simulink model "SSM"  (R2022b)
settings: configuration reference "ERT" (kept outside this file)
undefined symbols (not defined in the file): bIsCtl_P, cntPreFailrPerm_C, CodeChkOfsCal_C, DFC, ECM, EiceSilSM, FID, flgIgrDfc_C, nHystFwlAsc_C, nTransFwlAsc_C, Ts_10ms, ubrMax_C, ubrMin_C, uDcLinkPreChrg_C, uThdUmax_C, uThdURng1_C, uThdURng1Hyst_C, uThdURng3Hyst_C
libraries: simulink x8, DSMLib x8
settings Model: Creator=M00039784  LastModifiedBy=M00039784
settings ConfigSetRef: SourceName=ERT  SourceLocation=Base Workspace

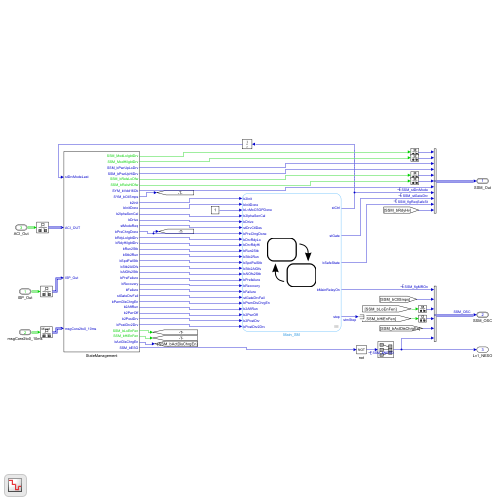
[thumbnail: Simulink's stored preview of the top-level diagram]
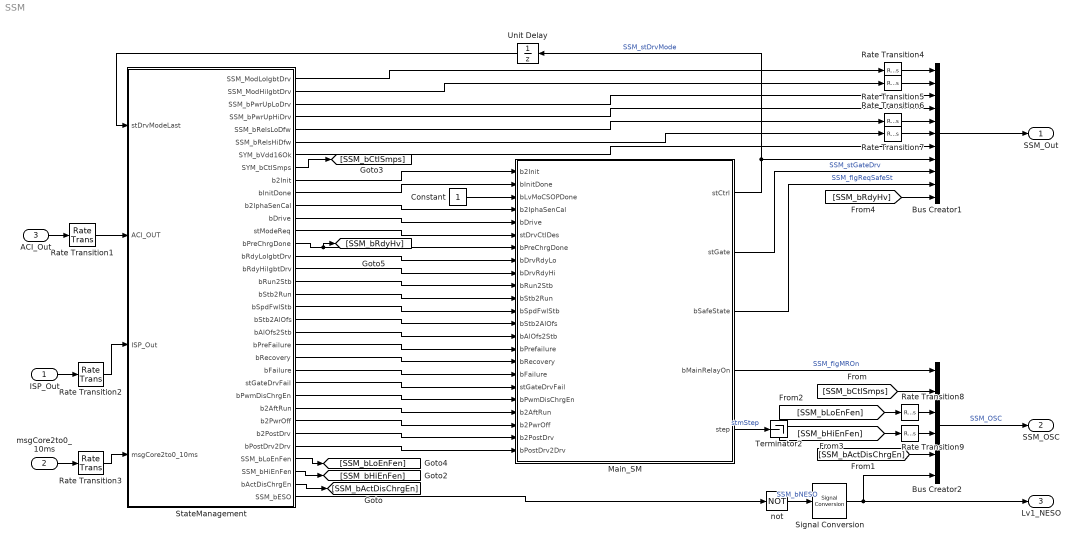
== system SSM ==
  ISP_Out : Inport  OutDataTypeStr=Bus: Core0_ISP_Out
  msgCore2to0_10ms : Inport  Port=2  OutDataTypeStr=Bus: Sig10ms20ST
  ACI_Out : Inport  Port=3  OutDataTypeStr=Bus: IO_In_1ms
  Bus Creator1 : BusCreator  Inputs=11  OutDataTypeStr=Bus: Core0_SSM_Out
  Bus Creator2 : BusCreator  Inputs=6  OutDataTypeStr=Bus: Core0_SSM_OSC
  Constant : Constant  OutDataTypeStr=boolean
  Main_SM : Stateflow chart  Priority=0  TreatAsAtomicUnit=on  SystemSampleTime=Ts_10ms
  Rate Transition{1..9} (9 alike) : RateTransition  OutPortSampleTime=Ts_10ms
  Signal Conversion : SignalConversion  OverrideOpt=off
  StateManagement : Subsystem
  Terminator2 : Terminator
  Unit Delay : UnitDelay  InitialCondition=ECM.Init  SampleTime=-1  HasFrameUpgradeWarning=on
  not : Logic  Operator=NOT  AllPortsSameDT=off  OutDataTypeStr=boolean
  SSM_Out : Outport  OutDataTypeStr=Bus: Core0_SSM_Out  VectorParamsAs1DForOutWhenUnconnected=off
  SSM_OSC : Outport  Port=2  OutDataTypeStr=Bus: Core0_SSM_OSC  VectorParamsAs1DForOutWhenUnconnected=off
  Lv1_NESO : Outport  Port=3  VectorParamsAs1DForOutWhenUnconnected=off
  wires:
  [SSM_bHiEnFen] -> Rate Transition9/1
  Rate Transition6/1 -> Bus Creator1/5
  [SSM_bCtlSmps] -> Bus Creator2/2
  Rate Transition7/1 -> Bus Creator1/6
  StateManagement/33(bActDisChrgEn) -> [SSM_bActDisChrgEn]
  StateManagement/21(bAlOfs2Stb) -> Main_SM/14(bAlOfs2Stb)
  StateManagement/17(bRun2Stb) -> Main_SM/10(bRun2Stb)
  Main_SM/4(bMainRelayOn) -> Bus Creator2/1  "SSM_flgMROn"
  Rate Transition9/1 -> Bus Creator2/4
  Main_SM/5(step) -> Terminator2/1  "stmStep"
  StateManagement/7(SYM_bVdd16Ok) -> Bus Creator1/7
  StateManagement/18(bStb2Run) -> Main_SM/11(bStb2Run)
  StateManagement/25(stGateDrvFail) -> Main_SM/18(stGateDrvFail)
  StateManagement/14(bPreChrgDone) -> [SSM_bRdyHv], Main_SM/7(bPreChrgDone)
  StateManagement/30(bPostDrv2Drv) -> Main_SM/23(bPostDrv2Drv)
  StateManagement/12(bDrive) -> Main_SM/5(bDrive)
  Rate Transition3/1 -> StateManagement/4(msgCore2to0_10ms)
  StateManagement/22(bPreFailure) -> Main_SM/15(bPrefailure)
  Main_SM/3(bSafeState) -> Bus Creator1/10  "SSM_flgReqSafeSt"
  StateManagement/1(SSM_ModLoIgbtDrv) -> Rate Transition4/1
  StateManagement/19(bSpdFwlStb) -> Main_SM/12(bSpdFwlStb)
  Rate Transition1/1 -> StateManagement/2(ACI_OUT)
  StateManagement/31(SSM_bLoEnFen) -> [SSM_bLoEnFen]
  Rate Transition4/1 -> Bus Creator1/1
  StateManagement/9(b2Init) -> Main_SM/1(b2Init)
  StateManagement/24(bFailure) -> Main_SM/17(bFailure)
  StateManagement/28(b2PwrOff) -> Main_SM/21(b2PwrOff)
  ISP_Out/1 -> Rate Transition2/1
  Bus Creator2/1 -> SSM_OSC/1  "SSM_OSC"
  StateManagement/29(b2PostDrv) -> Main_SM/22(b2PostDrv)
  StateManagement/11(b2IphaSenCal) -> Main_SM/4(b2IphaSenCal)
  ACI_Out/1 -> Rate Transition1/1
  Rate Transition5/1 -> Bus Creator1/2
  StateManagement/20(bStb2AlOfs) -> Main_SM/13(bStb2AlOfs)
  StateManagement/16(bRdyHiIgbtDrv) -> Main_SM/9(bDrvRdyHi)
  Bus Creator1/1 -> SSM_Out/1
  Constant/1 -> Main_SM/3(bLvMoCSOPDone)
  StateManagement/5(SSM_bRelsLoDfw) -> Rate Transition6/1
  Rate Transition2/1 -> StateManagement/3(ISP_Out)
  Main_SM/1(stCtrl) -> Unit Delay/1, Bus Creator1/8  "SSM_stDrvMode"
  StateManagement/15(bRdyLoIgbtDrv) -> Main_SM/8(bDrvRdyLo)
  StateManagement/27(b2AftRun) -> Main_SM/20(b2AftRun)
  StateManagement/2(SSM_ModHiIgbtDrv) -> Rate Transition5/1
  [SSM_bLoEnFen] -> Rate Transition8/1
  [SSM_bRdyHv] -> Bus Creator1/11
  StateManagement/8(SYM_bCtlSmps) -> [SSM_bCtlSmps]
  msgCore2to0_10ms/1 -> Rate Transition3/1
  Unit Delay/1 -> StateManagement/1(stDrvModeLast)
  Rate Transition8/1 -> Bus Creator2/3
  StateManagement/23(bRecovery) -> Main_SM/16(bRecovery)
  not/1 -> Signal Conversion/1  "SSM_bNESO"
  StateManagement/32(SSM_bHiEnFen) -> [SSM_bHiEnFen]
  StateManagement/10(bInitDone) -> Main_SM/2(bInitDone)
  [SSM_bActDisChrgEn] -> Bus Creator2/5
  StateManagement/3(SSM_bPwrUpLoDrv) -> Bus Creator1/3
  StateManagement/13(stModeReq) -> Main_SM/6(stDrvCtlDes)
  StateManagement/34(SSM_bESO) -> not/1
  StateManagement/6(SSM_bRelsHiDfw) -> Rate Transition7/1
  StateManagement/4(SSM_bPwrUpHiDrv) -> Bus Creator1/4
  Main_SM/2(stGate) -> Bus Creator1/9  "SSM_stGateDrv"
  StateManagement/26(bPwmDisChrgEn) -> Main_SM/19(bPwmDisChrgEn)
  Signal Conversion/1 -> Lv1_NESO/1, Bus Creator2/6

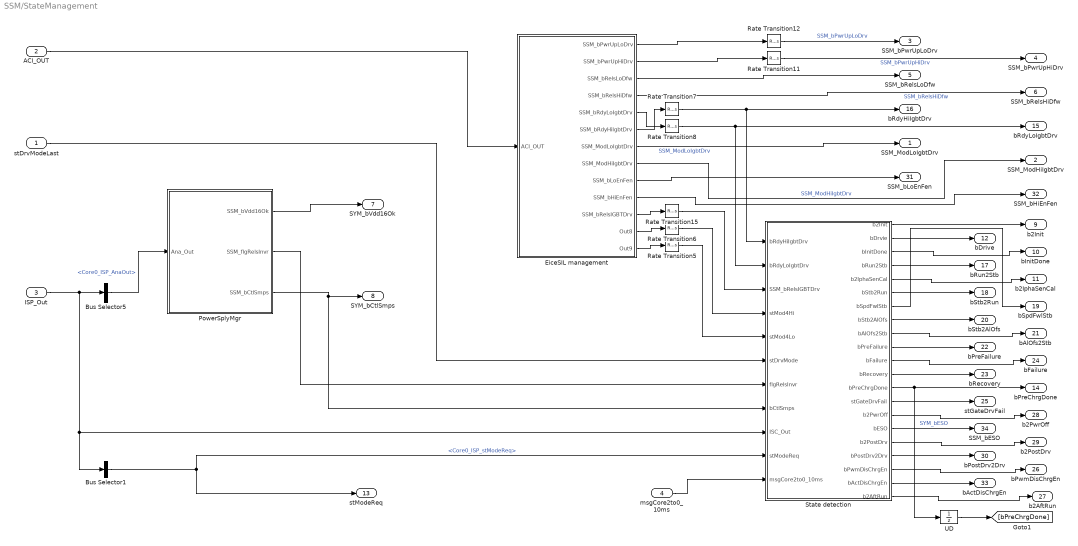
== system SSM/StateManagement ==
  stDrvModeLast : Inport
  ACI_OUT : Inport  Port=2  OutDataTypeStr=Bus: IO_In_1ms
  ISP_Out : Inport  Port=3
  msgCore2to0_10ms : Inport  Port=4
  Bus Selector1 : BusSelector  OutputSignals=Core0_ISP_ComCmd.Core0_ISP_stModeReq
  Bus Selector5 : BusSelector  OutputSignals=Core0_ISP_AnaOut
  EiceSIL management : Subsystem
  PowerSplyMgr : Subsystem
  Rate Transition{5..8,11..12,15} (7 alike) : RateTransition  OutPortSampleTime=Ts_10ms
  State detection : Subsystem
  UD : UnitDelay  SampleTime=-1  HasFrameUpgradeWarning=on
  SSM_ModLoIgbtDrv : Outport  VectorParamsAs1DForOutWhenUnconnected=off
  SSM_ModHiIgbtDrv : Outport  Port=2  VectorParamsAs1DForOutWhenUnconnected=off
  SSM_bPwrUpLoDrv : Outport  Port=3  VectorParamsAs1DForOutWhenUnconnected=off
  SSM_bPwrUpHiDrv : Outport  Port=4  VectorParamsAs1DForOutWhenUnconnected=off
  SSM_bRelsLoDfw : Outport  Port=5  VectorParamsAs1DForOutWhenUnconnected=off
  SSM_bRelsHiDfw : Outport  Port=6  VectorParamsAs1DForOutWhenUnconnected=off
  SYM_bVdd16Ok : Outport  Port=7  VectorParamsAs1DForOutWhenUnconnected=off
  SYM_bCtlSmps : Outport  Port=8  VectorParamsAs1DForOutWhenUnconnected=off
  b2Init : Outport  Port=9  VectorParamsAs1DForOutWhenUnconnected=off
  bInitDone : Outport  Port=10  VectorParamsAs1DForOutWhenUnconnected=off
  b2IphaSenCal : Outport  Port=11  VectorParamsAs1DForOutWhenUnconnected=off
  bDrive : Outport  Port=12  VectorParamsAs1DForOutWhenUnconnected=off
  stModeReq : Outport  Port=13  VectorParamsAs1DForOutWhenUnconnected=off
  bPreChrgDone : Outport  Port=14  VectorParamsAs1DForOutWhenUnconnected=off
  bRdyLoIgbtDrv : Outport  Port=15  VectorParamsAs1DForOutWhenUnconnected=off
  bRdyHiIgbtDrv : Outport  Port=16  VectorParamsAs1DForOutWhenUnconnected=off
  bRun2Stb : Outport  Port=17  VectorParamsAs1DForOutWhenUnconnected=off
  bStb2Run : Outport  Port=18  VectorParamsAs1DForOutWhenUnconnected=off
  bSpdFwlStb : Outport  Port=19  VectorParamsAs1DForOutWhenUnconnected=off
  bStb2AlOfs : Outport  Port=20  VectorParamsAs1DForOutWhenUnconnected=off
  bAlOfs2Stb : Outport  Port=21  VectorParamsAs1DForOutWhenUnconnected=off
  bPreFailure : Outport  Port=22  VectorParamsAs1DForOutWhenUnconnected=off
  bRecovery : Outport  Port=23  VectorParamsAs1DForOutWhenUnconnected=off
  bFailure : Outport  Port=24  VectorParamsAs1DForOutWhenUnconnected=off
  stGateDrvFail : Outport  Port=25  VectorParamsAs1DForOutWhenUnconnected=off
  bPwmDisChrgEn : Outport  Port=26  VectorParamsAs1DForOutWhenUnconnected=off
  b2AftRun : Outport  Port=27  VectorParamsAs1DForOutWhenUnconnected=off
  b2PwrOff : Outport  Port=28  VectorParamsAs1DForOutWhenUnconnected=off
  b2PostDrv : Outport  Port=29  VectorParamsAs1DForOutWhenUnconnected=off
  bPostDrv2Drv : Outport  Port=30  VectorParamsAs1DForOutWhenUnconnected=off
  SSM_bLoEnFen : Outport  Port=31  VectorParamsAs1DForOutWhenUnconnected=off
  SSM_bHiEnFen : Outport  Port=32  VectorParamsAs1DForOutWhenUnconnected=off
  bActDisChrgEn : Outport  Port=33  VectorParamsAs1DForOutWhenUnconnected=off
  SSM_bESO : Outport  Port=34  VectorParamsAs1DForOutWhenUnconnected=off
  wires:
  Bus Selector5/1 -> PowerSplyMgr/1(Ana_Out)  "<Core0_ISP_AnaOut>"
  Bus Selector1/1 -> State detection/10(stModeReq), stModeReq/1  "<Core0_ISP_stModeReq>"
  ISP_Out/1 -> Bus Selector5/1, Bus Selector1/1, State detection/9(ISC_Out)
  PowerSplyMgr/3(SSM_bCtlSmps) -> State detection/8(bCtlSmps), SYM_bCtlSmps/1
  msgCore2to0_10ms/1 -> State detection/11(msgCore2to0_10ms)
  EiceSIL management/1(SSM_bPwrUpLoDrv) -> Rate Transition12/1
  EiceSIL management/2(SSM_bPwrUpHiDrv) -> Rate Transition11/1
  stDrvModeLast/1 -> State detection/6(stDrvMode)
  PowerSplyMgr/1(SSM_bVdd16Ok) -> SYM_bVdd16Ok/1
  EiceSIL management/9(SSM_bLoEnFen) -> SSM_bLoEnFen/1
  EiceSIL management/10(SSM_bHiEnFen) -> SSM_bHiEnFen/1
  State detection/13(bPreChrgDone) -> UD/1, bPreChrgDone/1
  State detection/4(bRun2Stb) -> bRun2Stb/1
  State detection/6(bStb2Run) -> bStb2Run/1
  State detection/7(bSpdFwlStb) -> bSpdFwlStb/1
  State detection/8(bStb2AlOfs) -> bStb2AlOfs/1
  State detection/9(bAlOfs2Stb) -> bAlOfs2Stb/1
  State detection/10(bPreFailure) -> bPreFailure/1
  State detection/12(bRecovery) -> bRecovery/1
  State detection/11(bFailure) -> bFailure/1
  State detection/3(bInitDone) -> bInitDone/1
  State detection/2(bDrvie) -> bDrive/1
  EiceSIL management/12(Out8) -> Rate Transition6/1
  Rate Transition5/1 -> State detection/5(stMod4Lo)
  Rate Transition6/1 -> State detection/4(stMod4Hi)
  EiceSIL management/6(SSM_bRdyHiIgbtDrv) -> Rate Transition7/1
  EiceSIL management/5(SSM_bRdyLoIgbtDrv) -> Rate Transition8/1
  EiceSIL management/4(SSM_bRelsHiDfw) -> SSM_bRelsHiDfw/1  "SSM_bRelsHiDfw"
  Rate Transition11/1 -> SSM_bPwrUpHiDrv/1  "SSM_bPwrUpHiDrv"
  Rate Transition12/1 -> SSM_bPwrUpLoDrv/1  "SSM_bPwrUpLoDrv"
  Rate Transition7/1 -> bRdyHiIgbtDrv/1, State detection/1(bRdyHiIgbtDrv)
  Rate Transition8/1 -> bRdyLoIgbtDrv/1, State detection/2(bRdyLoIgbtDrv)
  EiceSIL management/7(SSM_ModLoIgbtDrv) -> SSM_ModLoIgbtDrv/1  "SSM_ModLoIgbtDrv"
  EiceSIL management/8(SSM_ModHiIgbtDrv) -> SSM_ModHiIgbtDrv/1  "SSM_ModHiIgbtDrv"
  ACI_OUT/1 -> EiceSIL management/1(ACI_OUT)
  EiceSIL management/11(SSM_bRelsIGBTDrv) -> Rate Transition15/1
  Rate Transition15/1 -> State detection/3(SSM_bRelsIGBTDrv)
  UD/1 -> [bPreChrgDone]
  PowerSplyMgr/2(SSM_flgRelsInvr) -> State detection/7(flgRelsInvr)
  State detection/14(stGateDrvFail) -> stGateDrvFail/1
  State detection/16(bESO) -> SSM_bESO/1  "SYM_bESO"
  State detection/5(b2IphaSenCal) -> b2IphaSenCal/1
  State detection/1(b2Init) -> b2Init/1
  State detection/17(b2PostDrv) -> b2PostDrv/1
  State detection/18(bPostDrv2Drv) -> bPostDrv2Drv/1
  State detection/21(b2AftRun) -> b2AftRun/1
  State detection/19(bPwmDisChrgEn) -> bPwmDisChrgEn/1
  State detection/15(b2PwrOff) -> b2PwrOff/1
  State detection/20(bActDisChrgEn) -> bActDisChrgEn/1
  EiceSIL management/13(Out9) -> Rate Transition5/1
  EiceSIL management/3(SSM_bRelsLoDfw) -> SSM_bRelsLoDfw/1

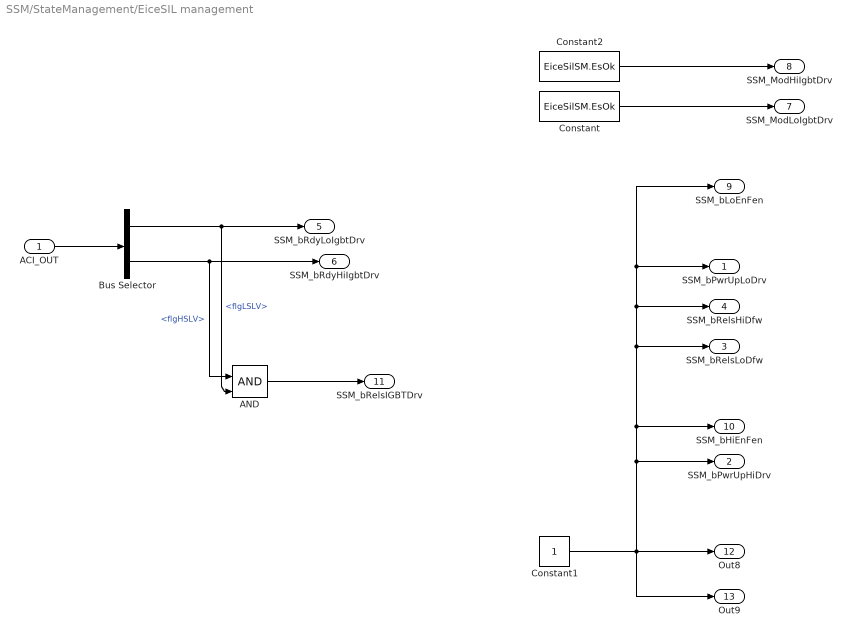
== system SSM/StateManagement/EiceSIL management ==
  ACI_OUT : Inport
  AND : Logic  IconShape=distinctive  AllPortsSameDT=off  OutDataTypeStr=boolean
  Bus Selector : BusSelector  OutputSignals=flgLSLV,flgHSLV
  Constant : Constant  Value=EiceSilSM.EsOk
  Constant1 : Constant  OutDataTypeStr=boolean
  Constant2 : Constant  Value=EiceSilSM.EsOk
  SSM_bPwrUpLoDrv : Outport
  SSM_bPwrUpHiDrv : Outport  Port=2
  SSM_bRelsLoDfw : Outport  Port=3
  SSM_bRelsHiDfw : Outport  Port=4
  SSM_bRdyLoIgbtDrv : Outport  Port=5  VectorParamsAs1DForOutWhenUnconnected=off
  SSM_bRdyHiIgbtDrv : Outport  Port=6  VectorParamsAs1DForOutWhenUnconnected=off
  SSM_ModLoIgbtDrv : Outport  Port=7  VectorParamsAs1DForOutWhenUnconnected=off
  SSM_ModHiIgbtDrv : Outport  Port=8  VectorParamsAs1DForOutWhenUnconnected=off
  SSM_bLoEnFen : Outport  Port=9  VectorParamsAs1DForOutWhenUnconnected=off
  SSM_bHiEnFen : Outport  Port=10  VectorParamsAs1DForOutWhenUnconnected=off
  SSM_bRelsIGBTDrv : Outport  Port=11  VectorParamsAs1DForOutWhenUnconnected=off
  Out8 : Outport  Port=12
  Out9 : Outport  Port=13
  wires:
  Constant/1 -> SSM_ModLoIgbtDrv/1
  Constant1/1 -> SSM_bPwrUpHiDrv/1, SSM_bRelsLoDfw/1, SSM_bRelsHiDfw/1, SSM_bPwrUpLoDrv/1, SSM_bLoEnFen/1, SSM_bHiEnFen/1, Out9/1, Out8/1
  ACI_OUT/1 -> Bus Selector/1
  Bus Selector/1 -> AND/2, SSM_bRdyLoIgbtDrv/1  "<flgLSLV>"
  Bus Selector/2 -> SSM_bRdyHiIgbtDrv/1, AND/1  "<flgHSLV>"
  AND/1 -> SSM_bRelsIGBTDrv/1
  Constant2/1 -> SSM_ModHiIgbtDrv/1

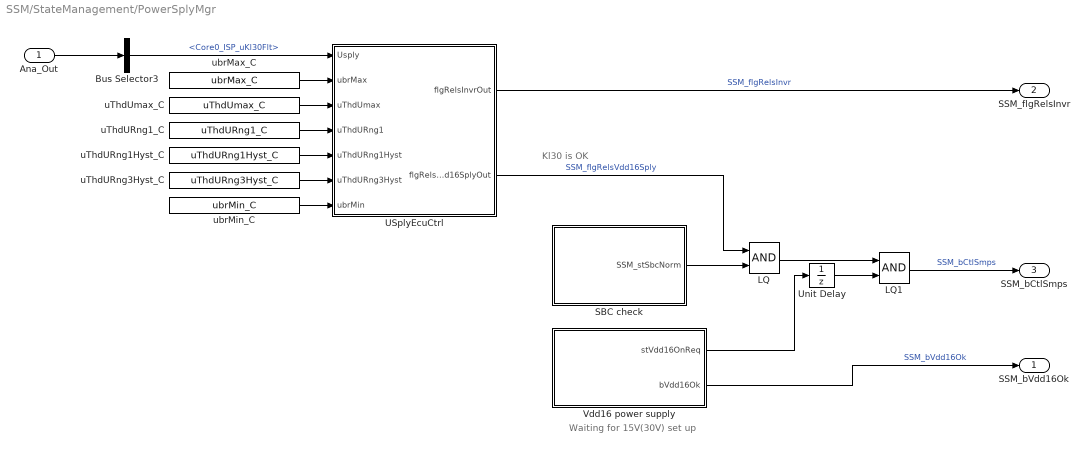
== system SSM/StateManagement/PowerSplyMgr ==
  note: Waiting for 15V(30V) set up
  note: Kl30 is OK
  Ana_Out : Inport
  Bus Selector3 : BusSelector  OutputSignals=Core0_ISP_uKl30Flt
  LQ : Logic  AllPortsSameDT=off  OutDataTypeStr=boolean
  LQ1 : Logic  AllPortsSameDT=off  OutDataTypeStr=boolean
  SBC check : Subsystem
  USplyEcuCtrl : MATLAB Function
  Unit Delay : UnitDelay  InitialCondition=false  SampleTime=-1  HasFrameUpgradeWarning=on
  Vdd16 power supply : Subsystem
  uThdURng1Hyst_C : Constant  Value=uThdURng1Hyst_C
      mask Display:
      | tmpx = get_param(gcbh,'Value');
      | a= evalin('base',[tmpx,'.Value;']);
      | disp([tmpx,': ',num2str(a)]);
  uThdURng1_C : Constant  Value=uThdURng1_C
      mask Display:
      | tmpx = get_param(gcbh,'Value');
      | a= evalin('base',[tmpx,'.Value;']);
      | disp([tmpx,': ',num2str(a)]);
  uThdURng3Hyst_C : Constant  Value=uThdURng3Hyst_C
      mask Display:
      | tmpx = get_param(gcbh,'Value');
      | a= evalin('base',[tmpx,'.Value;']);
      | disp([tmpx,': ',num2str(a)]);
  uThdUmax_C : Constant  Value=uThdUmax_C
      mask Display:
      | tmpx = get_param(gcbh,'Value');
      | a= evalin('base',[tmpx,'.Value;']);
      | disp([tmpx,': ',num2str(a)]);
  ubrMax_C : Constant  Value=ubrMax_C
      mask Display:
      | tmpx = get_param(gcbh,'Value');
      | a= evalin('base',[tmpx,'.Value;']);
      | disp([tmpx,': ',num2str(a)]);
  ubrMin_C : Constant  Value=ubrMin_C
      mask Display:
      | tmpx = get_param(gcbh,'Value');
      | a= evalin('base',[tmpx,'.Value;']);
      | disp([tmpx,': ',num2str(a)]);
  SSM_bVdd16Ok : Outport  VectorParamsAs1DForOutWhenUnconnected=off
  SSM_flgRelsInvr : Outport  Port=2  VectorParamsAs1DForOutWhenUnconnected=off
  SSM_bCtlSmps : Outport  Port=3  VectorParamsAs1DForOutWhenUnconnected=off
  wires:
  Ana_Out/1 -> Bus Selector3/1
  Bus Selector3/1 -> USplyEcuCtrl/1(Usply)  "<Core0_ISP_uKl30Flt>"
  USplyEcuCtrl/1(flgRelsInvrOut) -> SSM_flgRelsInvr/1  "SSM_flgRelsInvr"
  USplyEcuCtrl/2(flgRelsVdd16SplyOut) -> LQ/1  "SSM_flgRelsVdd16Sply"
  SBC check/1(SSM_stSbcNorm) -> LQ/2
  Vdd16 power supply/2(bVdd16Ok) -> SSM_bVdd16Ok/1  "SSM_bVdd16Ok"
  ubrMax_C/1 -> USplyEcuCtrl/2(ubrMax)
  uThdUmax_C/1 -> USplyEcuCtrl/3(uThdUmax)
  uThdURng1_C/1 -> USplyEcuCtrl/4(uThdURng1)
  uThdURng1Hyst_C/1 -> USplyEcuCtrl/5(uThdURng1Hyst)
  uThdURng3Hyst_C/1 -> USplyEcuCtrl/6(uThdURng3Hyst)
  ubrMin_C/1 -> USplyEcuCtrl/7(ubrMin)
  LQ/1 -> LQ1/1
  Vdd16 power supply/1(stVdd16OnReq) -> Unit Delay/1
  Unit Delay/1 -> LQ1/2
  LQ1/1 -> SSM_bCtlSmps/1  "SSM_bCtlSmps"

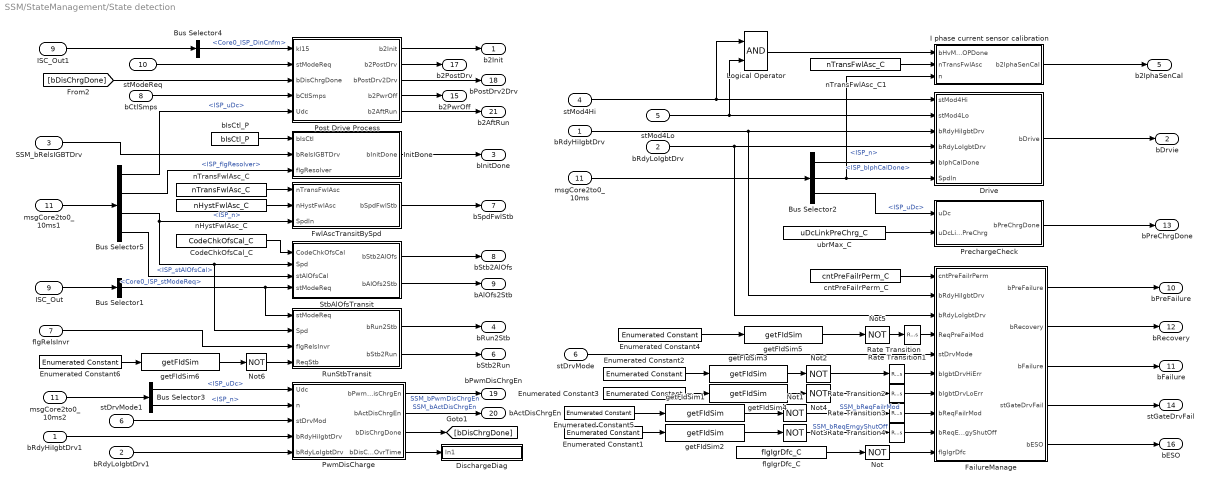
== system SSM/StateManagement/State detection ==
  bRdyHiIgbtDrv : Inport
  bRdyLoIgbtDrv : Inport  Port=2
  SSM_bRelsIGBTDrv : Inport  Port=3
  stMod4Hi : Inport  Port=4
  stMod4Lo : Inport  Port=5
  stDrvMode : Inport  Port=6
  flgRelsInvr : Inport  Port=7
  bCtlSmps : Inport  Port=8
  ISC_Out : Inport  Port=9
  stModeReq : Inport  Port=10
  msgCore2to0_10ms : Inport  Port=11
  Bus Selector1 : BusSelector  OutputSignals=Core0_ISP_ComCmd.Core0_ISP_stModeReq
  Bus Selector2 : BusSelector  OutputSignals=ISP_bIphCalDone,ISP_n,ISP_uDc
  Bus Selector3 : BusSelector  OutputSignals=ISP_uDc,ISP_n
  Bus Selector4 : BusSelector  OutputSignals=Core0_ISP_DinCnfm
  Bus Selector5 : BusSelector  OutputSignals=ISP_uDc,ISP_flgResolver,ISP_n,ISP_stAlOfsCal
  CodeChkOfsCal_C : Constant  Value=CodeChkOfsCal_C
      mask Display:
      | tmpx = get_param(gcbh,'Value');
      | a= evalin('base',[tmpx,'.Value;']);
      | disp([tmpx,': ',num2str(a)]);
  DischargeDiag : Subsystem
  Drive : MATLAB Function
  Enumerated Constant1 : simulink/Sources/Enumerated Constant  OutDataTypeStr=Enum: FID  Value=FID.ReqEmgyShutOff  SampleTime=inf
  Enumerated Constant2 : simulink/Sources/Enumerated Constant  OutDataTypeStr=Enum: FID  Value=FID.ReqIgbtDrvHiInvld  SampleTime=inf
  Enumerated Constant3 : simulink/Sources/Enumerated Constant  OutDataTypeStr=Enum: FID  Value=FID.ReqIgbtDrvLoInvld  SampleTime=inf
  Enumerated Constant4 : simulink/Sources/Enumerated Constant  OutDataTypeStr=Enum: FID  Value=FID.ReqPreFaiMod  SampleTime=inf
  Enumerated Constant5 : simulink/Sources/Enumerated Constant  OutDataTypeStr=Enum: FID  Value=FID.ReqFailrMod  SampleTime=inf
  Enumerated Constant6 : simulink/Sources/Enumerated Constant  OutDataTypeStr=Enum: FID  Value=FID.ReqStandby  SampleTime=inf
  FailureManage : MATLAB Function
  FwlAscTransitBySpd : MATLAB Function
  I phase current sensor calibration : MATLAB Function
  ISC_Out1 : InportShadow  Port=9
  InitDone : MATLAB Function
  Logical Operator : Logic  AllPortsSameDT=off  OutDataTypeStr=boolean
  Not{,1..6} (7 alike) : Logic  Operator=NOT  AllPortsSameDT=off  OutDataTypeStr=boolean
  Post Drive Process : MATLAB Function
  PrechargeCheck : MATLAB Function
  PwmDisCharge : MATLAB Function
  Rate Transition{,1..4} (5 alike) : RateTransition  OutPortSampleTime=Ts_10ms
  RunStbTransit : MATLAB Function
  StbAlOfsTransit : MATLAB Function
  bIsCtl_P : Constant  Value=bIsCtl_P
      mask Display:
      | tmpx = get_param(gcbh,'Value');
      | a= evalin('base',[tmpx,'.Value;']);
      | disp([tmpx,': ',num2str(a)]);
  bRdyHiIgbtDrv1 : InportShadow
  bRdyLoIgbtDrv1 : InportShadow  Port=2
  cntPreFailrPerm_C : Constant  Value=cntPreFailrPerm_C
      mask Display:
      | tmpx = get_param(gcbh,'Value');
      | a= evalin('base',[tmpx,'.Value;']);
      | disp([tmpx,': ',num2str(a)]);
  flgIgrDfc_C : Constant  Value=flgIgrDfc_C
      mask Display:
      | tmpx = get_param(gcbh,'Value');
      | a= evalin('base',[tmpx,'.Value;']);
      | disp([tmpx,': ',num2str(a)]);
  getFIdSim{1..6} (6 alike) : DSMLib/getFIdSim  SystemSampleTime=-1  VariantActivationTime=update diagram  Latency=0  AutoFrameSizeCalculation=off
  msgCore2to0_10ms1 : InportShadow  Port=11
  msgCore2to0_10ms2 : InportShadow  Port=11
  nHystFwlAsc_C : Constant  Value=nHystFwlAsc_C
      mask Display:
      | tmpx = get_param(gcbh,'Value');
      | a= evalin('base',[tmpx,'.Value;']);
      | disp([tmpx,': ',num2str(a)]);
  nTransFwlAsc_C : Constant  Value=nTransFwlAsc_C
      mask Display:
      | tmpx = get_param(gcbh,'Value');
      | a= evalin('base',[tmpx,'.Value;']);
      | disp([tmpx,': ',num2str(a)]);
  nTransFwlAsc_C1 : Constant  Value=nTransFwlAsc_C
      mask Display:
      | tmpx = get_param(gcbh,'Value');
      | a= evalin('base',[tmpx,'.Value;']);
      | disp([tmpx,': ',num2str(a)]);
  stDrvMode1 : InportShadow  Port=6
  ubrMax_C : Constant  Value=uDcLinkPreChrg_C
      mask Display:
      | tmpx = get_param(gcbh,'Value');
      | a= evalin('base',[tmpx,'.Value;']);
      | disp([tmpx,': ',num2str(a)]);
  b2Init : Outport  VectorParamsAs1DForOutWhenUnconnected=off
  bDrvie : Outport  Port=2  VectorParamsAs1DForOutWhenUnconnected=off
  bInitDone : Outport  Port=3  VectorParamsAs1DForOutWhenUnconnected=off
  bRun2Stb : Outport  Port=4  VectorParamsAs1DForOutWhenUnconnected=off
  b2IphaSenCal : Outport  Port=5  VectorParamsAs1DForOutWhenUnconnected=off
  bStb2Run : Outport  Port=6  VectorParamsAs1DForOutWhenUnconnected=off
  bSpdFwlStb : Outport  Port=7  VectorParamsAs1DForOutWhenUnconnected=off
  bStb2AlOfs : Outport  Port=8  VectorParamsAs1DForOutWhenUnconnected=off
  bAlOfs2Stb : Outport  Port=9  VectorParamsAs1DForOutWhenUnconnected=off
  bPreFailure : Outport  Port=10  VectorParamsAs1DForOutWhenUnconnected=off
  bFailure : Outport  Port=11  VectorParamsAs1DForOutWhenUnconnected=off
  bRecovery : Outport  Port=12  VectorParamsAs1DForOutWhenUnconnected=off
  bPreChrgDone : Outport  Port=13  VectorParamsAs1DForOutWhenUnconnected=off
  stGateDrvFail : Outport  Port=14  VectorParamsAs1DForOutWhenUnconnected=off
  b2PwrOff : Outport  Port=15  VectorParamsAs1DForOutWhenUnconnected=off
  bESO : Outport  Port=16  VectorParamsAs1DForOutWhenUnconnected=off
  b2PostDrv : Outport  Port=17  VectorParamsAs1DForOutWhenUnconnected=off
  bPostDrv2Drv : Outport  Port=18  VectorParamsAs1DForOutWhenUnconnected=off
  bPwmDisChrgEn : Outport  Port=19  VectorParamsAs1DForOutWhenUnconnected=off
  bActDisChrgEn : Outport  Port=20  VectorParamsAs1DForOutWhenUnconnected=off
  b2AftRun : Outport  Port=21  VectorParamsAs1DForOutWhenUnconnected=off
  wires:
  Bus Selector5/2 -> InitDone/3(flgResolver)  "<ISP_flgResolver>"
  StbAlOfsTransit/1(bStb2AlOfs) -> bStb2AlOfs/1
  StbAlOfsTransit/2(bAlOfs2Stb) -> bAlOfs2Stb/1
  FailureManage/1(bPreFailure) -> bPreFailure/1
  FailureManage/2(bRecovery) -> bRecovery/1
  FwlAscTransitBySpd/1(bSpdFwlStb) -> bSpdFwlStb/1
  RunStbTransit/2(bStb2Run) -> bStb2Run/1
  RunStbTransit/1(bRun2Stb) -> bRun2Stb/1
  Bus Selector2/3 -> PrechargeCheck/1(uDc)  "<ISP_uDc>"
  Bus Selector2/2 -> I phase current sensor calibration/3(n), Drive/6(SpdIn)  "<ISP_n>"
  bRdyHiIgbtDrv/1 -> FailureManage/2(bRdyHiIgbtDrv), Drive/3(bRdyHiIgbtDrv)
  PrechargeCheck/1(bPreChrgDone) -> bPreChrgDone/1
  Bus Selector2/1 -> Drive/5(bIphCalDone)  "<ISP_bIphCalDone>"
  InitDone/1(bInitDone) -> bInitDone/1
  msgCore2to0_10ms/1 -> Bus Selector2/1
  Bus Selector1/1 -> RunStbTransit/1(stModeReq), StbAlOfsTransit/4(stModeReq)  "<Core0_ISP_stModeReq>"
  stDrvMode/1 -> FailureManage/5(stDrvMode)
  ISC_Out/1 -> Bus Selector1/1
  bRdyLoIgbtDrv/1 -> Drive/4(bRdyLoIgbtDrv), FailureManage/3(bRdyLoIgbtDrv)
  Drive/1(bDrive) -> bDrvie/1
  stMod4Hi/1 -> Logical Operator/1, Drive/1(stMod4Hi)
  stMod4Lo/1 -> Drive/2(stMod4Lo), Logical Operator/2
  SSM_bRelsIGBTDrv/1 -> InitDone/2(bRelsIGBTDrv)
  FailureManage/4(stGateDrvFail) -> stGateDrvFail/1
  FailureManage/5(bESO) -> bESO/1
  Logical Operator/1 -> I phase current sensor calibration/1(bHvMoCSOPDone)
  flgRelsInvr/1 -> RunStbTransit/3(flgRelsInvr)
  msgCore2to0_10ms1/1 -> Bus Selector5/1
  Bus Selector5/3 -> RunStbTransit/2(Spd), StbAlOfsTransit/2(Spd), FwlAscTransitBySpd/3(SpdIn)  "<ISP_n>"
  Bus Selector5/4 -> StbAlOfsTransit/3(stAlOfsCal)  "<ISP_stAlOfsCal>"
  Enumerated Constant5/1 -> getFIdSim1/1
  flgIgrDfc_C/1 -> Not/1
  getFIdSim1/1 -> Not1/1
  Not1/1 -> Rate Transition3/1  "SSM_bReqFailrMod"
  Not/1 -> FailureManage/10(flgIgrDfc)
  FailureManage/3(bFailure) -> bFailure/1
  Enumerated Constant1/1 -> getFIdSim2/1
  getFIdSim2/1 -> Not3/1
  Not3/1 -> Rate Transition4/1  "SSM_bReqEmgyShutOff"
  Enumerated Constant2/1 -> getFIdSim3/1
  Enumerated Constant3/1 -> getFIdSim4/1
  getFIdSim3/1 -> Not2/1
  getFIdSim4/1 -> Not4/1
  Not2/1 -> Rate Transition1/1
  Not4/1 -> Rate Transition2/1
  Not5/1 -> Rate Transition/1
  getFIdSim5/1 -> Not5/1
  Enumerated Constant4/1 -> getFIdSim5/1
  cntPreFailrPerm_C/1 -> FailureManage/1(cntPreFailrPerm)
  getFIdSim6/1 -> Not6/1
  Enumerated Constant6/1 -> getFIdSim6/1
  Not6/1 -> RunStbTransit/4(ReqStb)
  ISC_Out1/1 -> Bus Selector4/1
  Post Drive Process/2(b2PostDrv) -> b2PostDrv/1
  msgCore2to0_10ms2/1 -> Bus Selector3/1
  PwmDisCharge/1(bPwmDisChrgEn) -> bPwmDisChrgEn/1  "SSM_bPwmDisChrgEn"
  Bus Selector3/1 -> PwmDisCharge/1(Udc)  "<ISP_uDc>"
  stDrvMode1/1 -> PwmDisCharge/3(stDrvMod)
  bRdyHiIgbtDrv1/1 -> PwmDisCharge/4(bRdyHiIgbtDrv)
  bRdyLoIgbtDrv1/1 -> PwmDisCharge/5(bRdyLoIgbtDrv)
  Bus Selector3/2 -> PwmDisCharge/2(n)  "<ISP_n>"
  PwmDisCharge/4(bDisChrgOvrTime) -> DischargeDiag/1(In1)
  Post Drive Process/1(b2Init) -> b2Init/1
  Post Drive Process/3(bPostDrv2Drv) -> bPostDrv2Drv/1
  Bus Selector4/1 -> Post Drive Process/1(kl15)  "<Core0_ISP_DinCnfm>"
  stModeReq/1 -> Post Drive Process/2(stModeReq)
  PwmDisCharge/3(bDisChrgDone) -> [bDisChrgDone]
  [bDisChrgDone] -> Post Drive Process/3(bDisChrgDone)
  I phase current sensor calibration/1(b2IphaSenCal) -> b2IphaSenCal/1
  nTransFwlAsc_C/1 -> FwlAscTransitBySpd/1(nTransFwlAsc)
  nHystFwlAsc_C/1 -> FwlAscTransitBySpd/2(nHystFwlAsc)
  nTransFwlAsc_C1/1 -> I phase current sensor calibration/2(nTransFwlAsc)
  Post Drive Process/4(b2PwrOff) -> b2PwrOff/1
  Post Drive Process/5(b2AftRun) -> b2AftRun/1
  bCtlSmps/1 -> Post Drive Process/4(bCtlSmps)
  ubrMax_C/1 -> PrechargeCheck/2(uDcLinkPreChrg)
  CodeChkOfsCal_C/1 -> StbAlOfsTransit/1(CodeChkOfsCal)
  PwmDisCharge/2(bActDisChrgEn) -> bActDisChrgEn/1  "SSM_bActDisChrgEn"
  Bus Selector5/1 -> Post Drive Process/5(Udc)  "<ISP_uDc>"
  bIsCtl_P/1 -> InitDone/1(bIsCtl)
  Rate Transition/1 -> FailureManage/4(ReqPreFaiMod)
  Rate Transition1/1 -> FailureManage/6(bIgbtDrvHiErr)
  Rate Transition2/1 -> FailureManage/7(bIgbtDrvLoErr)
  Rate Transition3/1 -> FailureManage/8(bReqFailrMod)
  Rate Transition4/1 -> FailureManage/9(bReqEmgyShutOff)

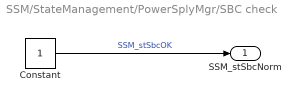
== system SSM/StateManagement/PowerSplyMgr/SBC check ==
  Constant : Constant  OutDataTypeStr=boolean
  SSM_stSbcNorm : Outport  VectorParamsAs1DForOutWhenUnconnected=off
  wires:
  Constant/1 -> SSM_stSbcNorm/1  "SSM_stSbcOK"

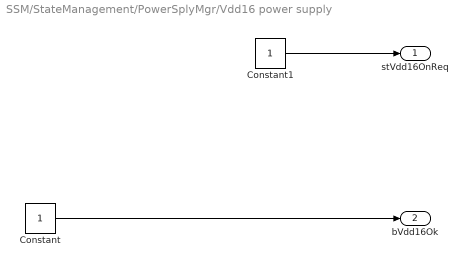
== system SSM/StateManagement/PowerSplyMgr/Vdd16 power supply ==
  Constant : Constant  OutDataTypeStr=boolean
  Constant1 : Constant  OutDataTypeStr=boolean
  stVdd16OnReq : Outport  VectorParamsAs1DForOutWhenUnconnected=off
  bVdd16Ok : Outport  Port=2  VectorParamsAs1DForOutWhenUnconnected=off
  wires:
  Constant/1 -> bVdd16Ok/1
  Constant1/1 -> stVdd16OnReq/1

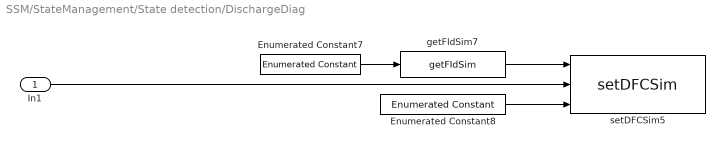
== system SSM/StateManagement/State detection/DischargeDiag ==
  In1 : Inport
  Enumerated Constant7 : simulink/Sources/Enumerated Constant  OutDataTypeStr=Enum: FID  Value=FID.DiagUdcDisChrg  SampleTime=inf
  Enumerated Constant8 : simulink/Sources/Enumerated Constant  OutDataTypeStr=Enum: DFC  Value=DFC.UdcDisChrgOvrTime  SampleTime=inf
  getFIdSim7 : DSMLib/getFIdSim  SystemSampleTime=-1  VariantActivationTime=update diagram  Latency=0  AutoFrameSizeCalculation=off
  setDFCSim5 : DSMLib/setDFCSim  SystemSampleTime=-1  VariantActivationTime=update diagram  Latency=0  AutoFrameSizeCalculation=off
  wires:
  In1/1 -> setDFCSim5/2
  Enumerated Constant7/1 -> getFIdSim7/1
  getFIdSim7/1 -> setDFCSim5/1
  Enumerated Constant8/1 -> setDFCSim5/3

== stateflow chart SSM/Main_SM ==
  state PreDrive
    en: %predrive init
    state State_PreInit
      en:step = 0;
      stCtrl = ECM.PreInit;
      bSafeState = true;
      stGate = EGM.Freewheel;
      bPreDrvDone = false;
    state State_Init
      en:step = 1;
      bSafeState = true;
      stCtrl = ECM.Init;
      stGate = EGM.Freewheel;
      bMainRelayOn = true; %MR on
    state State_LVMOCSOP
      en:step = 2;
      bSafeState = true;
      stCtrl =ECM.LvMoCSOP;
      %stGate defined in CddHwMgr
    state State_PREDRVDone
      en:step = 3;
      bSafeState = true;
      stCtrl =ECM.PreDrvDone;
      stGate = EGM.Freewheel;
      bPreDrvDone = true;
    (default) -> State_PreInit
    State_PreInit -> State_Init : [b2Init]
    State_Init -> State_LVMOCSOP : [bInitDone]
    State_LVMOCSOP -> State_PREDRVDone : [bLvMoCSOPDone]
  state PostDrive
    en: % postdrive init
    state State_Discharge
      en:step=11;
      stCtrl = ECM.Discharge;
      stGate = StASC(bDrvRdyLo,bDrvRdyHi);
      du:
      if bPwmDisChrgEn
      stGate = EGM.PWMDischarge;
      else
      stGate = StASC(bDrvRdyLo,bDrvRdyHi);
      end
    state State_PowerOff
      en:step=12;
      stCtrl = ECM.PowerOff;
      stGate = EGM.Freewheel;
    state State_Afterrun
      en:step=12;
      stCtrl = ECM.Afterrun;
      stGate = EGM.Freewheel;
      bMainRelayOn = false;
    (default) -> State_Discharge
    State_Discharge -> State_PowerOff : [b2PwrOff]
    State_PowerOff -> State_Afterrun : [b2AftRun]
  state Drive
    en:% drive init
    state State_Ready
      state State_Run
        en:step=9;
        [stCtrl,stGate] = StRun(stDrvCtlDes);
        du: [stCtrl,stGate] = StRun(stDrvCtlDes);
        ex: stGate = EGM.Freewheel
      state State_Standby
        en:
        step=7;
        bSafeState = false;
        stCtrl = ECM.Standby;
        if bSpdFwlStb
        stGate = EGM.Freewheel;
        else
        stGate = EGM.Freewheel;
        end
        du:
        if bSpdFwlStb
        stGate = EGM.Freewheel;
        else
        stGate = EGM.Freewheel;
        end
      state State_PreFailure
        en:step =10;
        stCtrl = ECM.PreFailure;
        stGate = EGM.Freewheel;
      state State_AlOfsDone
        en:step=8;
        stCtrl = ECM.alOfsCal;
        stGate = EGM.PWMRun;
      State_Run -> State_Standby [order 1] : [bRun2Stb]
      State_Standby -> State_Run [order 1] : [bStb2Run]
      State_Run -> State_PreFailure [order 2] : [bPrefailure]
      (default) -> State_Standby
      State_PreFailure -> State_Standby : [bRecovery]
      State_Standby -> State_AlOfsDone [order 2] : [bStb2AlOfs]
      State_AlOfsDone -> State_Standby : [bAlOfs2Stb]
    state State_PreCharge
      en:step =4;
      bSafeState = true;
      stCtrl = ECM.PreCharge;
      stGate = EGM.Freewheel;
    state State_HVMOCSOP
      en:step =5;
      stCtrl = ECM.HvMoCSOP;
      %stGate defined in CddHwMgr
    state State_SenCal
      en:step =6;
      bSafeState = false;
      stCtrl = ECM.SensCal;
      stGate = EGM.Freewheel;
    (default) -> State_PreCharge
    State_PreCharge -> State_HVMOCSOP : [bPreChrgDone]
    State_HVMOCSOP -> State_SenCal : [b2IphaSenCal]
    State_SenCal -> State_Ready : [bDrive]
  note: Discharge: High voltage (Vdc Link) discharge
      |
      | PwrOff: Low voltage side and IGBT driver power off.
  state State_Failure
    entry:step=12;
    bSafeState = true;
    stCtrl = ECM.Failure;
    stGate =stGateDrvFail;
  (default) -> PreDrive
  PreDrive -> PostDrive [order 1] : [b2PostDrv]
  PostDrive -> Drive : [bPostDrv2Drv]
  PreDrive -> Drive [order 2] : [bPreDrvDone]
  Drive -> PostDrive [order 1] : [b2PostDrv]
  State_Failure -> PostDrive : [b2PostDrv]
  Drive -> State_Failure [order 2] : [bFailure]
  data: des function_input; drv function_output; gate function_output; stIgbtDrvLo function_input; gate function_output; stIgbtDrvHi function_input; stCtrl output; stGate output; b2Init input; bInitDone input boolean; bLvMoCSOPDone input boolean; b2IphaSenCal input boolean; bDrive input boolean; stDrvCtlDes input Enum: ECM; bPreChrgDone input boolean; bDrvRdyLo input boolean; bDrvRdyHi input boolean; bRun2Stb input boolean; bStb2Run input; bSpdFwlStb input boolean; bSkipInit constant boolean =1; bSafeState output boolean; bMainRelayOn output boolean; step output; bStb2AlOfs input; bAlOfs2Stb input; bPrefailure input boolean; bRecovery input boolean; bFailure input boolean; stGateDrvFail input; bPwmDisChrgEn input; b2AftRun input boolean; b2PwrOff input; bPreDrvDone local boolean =false; b2PostDrv input; bPostDrv2Drv input
  function [drv,gate] = StRun(des):
    | function [drv,gate] = StRun(des)
    |     if (des == ECM.TrqCtrl) 
    |         drv = ECM.TrqCtrl;
    |         gate = EGM.PWMRun;
    |     elseif (des == ECM.nCtrl) 
    |         drv = ECM.nCtrl;
    |         gate = EGM.PWMRun;
    |     elseif (des == ECM.UdcCtrl) 
    |         drv = ECM.UdcCtrl;
    |         gate = EGM.PWMRun;
    |     elseif (des == ECM.IFCtrl) 
    |         drv = ECM.IFCtrl;
    |         gate = EGM.PWMRun;
    |     elseif (des == ECM.IsCtrl) 
    |     drv = ECM.IsCtrl;
    |     gate = EGM.PWMRun;
    |     else 
    |         drv = ECM.Standby;
    |         gate = EGM.Freewheel;
    |     end
  function gate  = StASC(stIgbtDrvLo,stIgbtDrvHi):
    | function gate  = StASC(stIgbtDrvLo,stIgbtDrvHi)
    | if (stIgbtDrvLo) 
    |     gate = EGM.Shortcircuit;
    | elseif (stIgbtDrvHi)
    |     gate = EGM.ShortcircuitTop;
    | else
    |     gate = EGM.Freewheel;
    | end

== matlab function SSM/StateManagement/State detection/InitDone ==
  data: bIsCtl input; bRelsIGBTDrv input; bInitDone output; flgResolver input
function bInitDone  = fcn(bIsCtl,bRelsIGBTDrv,flgResolver)
%
bInitDone = bRelsIGBTDrv&&(flgResolver==uint8(2)||bIsCtl);

== matlab function SSM/StateManagement/State detection/Drive ==
  data: stMod4Hi input; stMod4Lo input; bRdyHiIgbtDrv input; bDrive output; bRdyLoIgbtDrv input; bIphCalDone input; SpdIn input
function bDrive  = fcn(stMod4Hi,stMod4Lo,bRdyHiIgbtDrv,bRdyLoIgbtDrv,bIphCalDone,SpdIn)
%

if SpdIn<single(4000)
    if bIphCalDone==true
        bSenCalStb = true;
    else
        bSenCalStb = false;
    end
else
    bSenCalStb= true;
end

bDrive = bRdyHiIgbtDrv&&bRdyLoIgbtDrv&&stMod4Hi&&stMod4Lo&&bSenCalStb;

== matlab function SSM/StateManagement/State detection/PwmDisCharge ==
  data: Udc input; n input; bPwmDisChrgEn output; bActDisChrgEn output; stDrvMod input; bDisChrgDone output; bRdyHiIgbtDrv input; bRdyLoIgbtDrv input; bDisChrgOvrTime output
function [bPwmDisChrgEn,bActDisChrgEn,bDisChrgDone,bDisChrgOvrTime]  = fcn(Udc,n,stDrvMod,bRdyHiIgbtDrv,bRdyLoIgbtDrv)
%
persistent cntDisCharg;
persistent bDisChrgDoneTmp;
persistent bActDisChrgEnTmp;
persistent bDisChrgOvrTimeTmp;

if isempty(cntDisCharg)
    cntDisCharg = uint16(0);
    bDisChrgDoneTmp = false;
    bDisChrgOvrTimeTmp = false;
    bActDisChrgEnTmp = false;
end

if stDrvMod==ECM.Discharge
    cntDisCharg = cntDisCharg + uint16(1);
    
    if Udc<single(55) %<55V
        bDisChrgDoneTmp = true;
    else
        if bRdyHiIgbtDrv&&bRdyLoIgbtDrv&&(abs(n)<single(500))
            bActDisChrgEnTmp = true;
        else
            bActDisChrgEnTmp = false;
        end 
    end
    
    if cntDisCharg>uint16(200) %2s
        cntDisCharg = uint16(201);
        bActDisChrgEnTmp = false;
        bDisChrgOvrTimeTmp = true;
    end
else
    bActDisChrgEnTmp = false;
    bDisChrgDoneTmp = false;
    cntDisCharg = uint16(0);
end

bDisChrgDone = bDisChrgDoneTmp;
bActDisChrgEn = bActDisChrgEnTmp;
bPwmDisChrgEn = false;
bDisChrgOvrTime = bDisChrgOvrTimeTmp;

== matlab function SSM/StateManagement/PowerSplyMgr/USplyEcuCtrl ==
  data: Usply input; ubrMax input; uThdUmax input; flgRelsInvrOut output; uThdURng1 input; uThdURng1Hyst input; uThdURng3Hyst input; ubrMin input; flgRelsVdd16SplyOut output
function [flgRelsInvrOut,flgRelsVdd16SplyOut]  = fcn(Usply,ubrMax,uThdUmax,uThdURng1,uThdURng1Hyst,uThdURng3Hyst,ubrMin)
%
persistent tiDelta;
persistent tiURng1Actv;
persistent tiURng2Actv;
persistent tiURng3Actv;
persistent tiURng4Actv;
persistent flgURng1Actv;
persistent flgURng2Actv;
persistent flgURng3Actv;
persistent tiURng1Rcv_C;
persistent tiURng2Rcv_C;
persistent tiURng3Rcv_C;
persistent tiURng4Rcv_C;
persistent tiMaxRngC_C;
persistent flgRelsInvr;
persistent flgRelsVdd16Sply;

if isempty(tiDelta)
    tiDelta = single(0.01);
    tiURng1Actv = single(0);
    tiURng2Actv = single(0);
    tiURng3Actv = single(0);
    tiURng4Actv = single(0);
    flgURng1Actv = false;
    flgURng2Actv = false;
    flgURng3Actv = false;
    tiURng1Rcv_C = single(0.03);
    tiURng2Rcv_C = single(0.03);
    tiURng3Rcv_C = single(0.03);
    tiURng4Rcv_C = single(0.03);
    tiMaxRngC_C = single(3);
    flgRelsInvr = false;
    flgRelsVdd16Sply = false;
end

%URng1:9V~17V
if Usply>uThdUmax %17V, uThdUmax is about 17V, inverter will work in normal mode
    tiURng4Actv = tiURng4Actv + tiDelta;
    tiURng1Actv = tiURng1Actv - tiDelta;
    
    if tiURng4Actv>tiMaxRngC_C
            tiURng4Actv = tiMaxRngC_C;
    end
    
    if tiURng1Actv<single(0)
        tiURng1Actv = single(0);
    end
    
    flgURng1Actv = false;
else
    if Usply<(uThdUmax-uThdURng1Hyst)% about16.8V  inverter will work in normal mode
        tiURng4Actv = single(0);
        tiURng1Actv = tiURng1Actv + tiDelta;
        
        if tiURng1Actv>tiMaxRngC_C
            tiURng1Actv = tiMaxRngC_C;
        end
        
        flgURng1Actv = true;  %range 9V~17V is true
    end
end

%URng2:6V~9V
if Usply>uThdURng1 % >9V
    tiURng2Actv = tiURng2Actv - tiDelta;
    
    if tiURng2Actv<single(0)
        tiURng2Actv = single(0);
    end
    
    flgURng2Actv = false;
else
    if Usply<(uThdURng1-uThdURng1Hyst) % <8.8V
        tiURng1Actv = single(0);
        tiURng2Actv = tiURng2Actv + tiDelta;
        
        if tiURng2Actv>tiMaxRngC_C
            tiURng2Actv = tiMaxRngC_C;
        end
        
        flgURng2Actv = true;  %range 6V~8V is true
    end
end
    
%URng3:<5.8V
if Usply>(ubrMin+uThdURng3Hyst) % >6V
    tiURng3Actv = tiURng3Actv - tiDelta;
    
    if tiURng3Actv<single(0)
        tiURng3Actv = single(0);
    end
    
    flgURng3Actv = false;
else
    if Usply<ubrMin %5.8V
        tiURng2Actv = single(0);
        tiURng3Actv = tiURng3Actv + tiDelta;
        
        if tiURng3Actv>tiMaxRngC_C
            tiURng3Actv = tiMaxRngC_C;
        end
        
        flgURng3Actv = true;  %range <5.8 is true
    end
end
    
if (tiURng1Actv>tiURng1Rcv_C)&&flgURng1Actv&&(~flgURng2Actv)&&(~flgURng3Actv)
    flgRelsInvr = true;
    flgRelsVdd16Sply = true;
end

%>17V or 6~9V
if ((tiURng2Actv>tiURng2Rcv_C)&&flgURng2Actv&&(~flgURng3Actv))||((tiURng4Actv>tiURng4Rcv_C)&&(~flgURng1Actv))
    flgRelsInvr = false;
    flgRelsVdd16Sply = true;
end

if (Usply>ubrMax)||((tiURng3Actv>tiURng3Rcv_C)&&flgURng3Actv)  %Current maximum is about 22V
    flgRelsInvr = false;
    flgRelsVdd16Sply = false;
end

flgRelsInvrOut = flgRelsInvr;
flgRelsVdd16SplyOut = flgRelsVdd16Sply;

== matlab function SSM/StateManagement/State detection/Post Drive Process ==
  data: kl15 input; b2Init output; b2PostDrv output; bPostDrv2Drv output; stModeReq input; bDisChrgDone input; bCtlSmps input; Udc input; b2PwrOff output; b2AftRun output
function [b2Init,b2PostDrv,bPostDrv2Drv,b2PwrOff,b2AftRun]  = fcn(kl15,stModeReq,bDisChrgDone,bCtlSmps,Udc)
%
b2Init = kl15;
b2PostDrv = (~kl15)||(stModeReq==ECM.Discharge);
bPostDrv2Drv = false;
b2PwrOff = (~kl15)&&(bDisChrgDone||(Udc<single(55)));
b2AftRun = ~bCtlSmps;

== matlab function SSM/StateManagement/State detection/I phase current sensor calibration ==
  data: bHvMoCSOPDone input; nTransFwlAsc input; b2IphaSenCal output; n input
function b2IphaSenCal  = fcn(bHvMoCSOPDone,nTransFwlAsc,n)
%
b2IphaSenCal = bHvMoCSOPDone&&(abs(n)<nTransFwlAsc);

== matlab function SSM/StateManagement/State detection/FwlAscTransitBySpd ==
  data: nTransFwlAsc input; nHystFwlAsc input; SpdIn input; bSpdFwlStb output
function bSpdFwlStb  = fcn(nTransFwlAsc,nHystFwlAsc,SpdIn)
%
persistent flgSpdFwl;

if isempty(flgSpdFwl)
    flgSpdFwl = false;
end

if SpdIn<single(nTransFwlAsc)
    flgSpdFwl = false;
elseif SpdIn>single(nTransFwlAsc+nHystFwlAsc)
    flgSpdFwl = true;   
end

bSpdFwlStb = flgSpdFwl;

== matlab function SSM/StateManagement/State detection/RunStbTransit ==
  data: stModeReq input; Spd input; flgRelsInvr input; ReqStb input; bRun2Stb output; bStb2Run output
function [bRun2Stb,bStb2Run]  = fcn(stModeReq,Spd,flgRelsInvr,ReqStb)
%
nAbs = abs(Spd);
if ReqStb||nAbs>single(19000) %375
    bStb2Run = false;
    bRun2Stb = true;
else
    if ((stModeReq==ECM.TrqCtrl)||(stModeReq==ECM.nCtrl)||(stModeReq==ECM.IFCtrl)||(stModeReq==ECM.UdcCtrl)||(stModeReq==ECM.IsCtrl))...
       &&flgRelsInvr
        bStb2Run = true;
        bRun2Stb = false;
    else
        bStb2Run = false;
        bRun2Stb = true;
    end
end

== matlab function SSM/StateManagement/State detection/StbAlOfsTransit ==
  data: CodeChkOfsCal input; Spd input; stAlOfsCal input; stModeReq input; bStb2AlOfs output; bAlOfs2Stb output
function [bStb2AlOfs,bAlOfs2Stb]  = fcn(CodeChkOfsCal,Spd,stAlOfsCal,stModeReq)
%
%stAlOfsCal:
%0: Init or rotor position offset calibration processing
%1: Rotor position offset calibration successed
%2: Rotor position offset calibration failed
bStb2AlOfs = (stModeReq==ECM.alOfsCal)&&(stAlOfsCal==uint8(0))&&(Spd<single(100))&&(CodeChkOfsCal==uint32(12345678));

bAlOfs2Stb = (stModeReq==ECM.Standby)||((stAlOfsCal~=uint8(0))&&(Spd<single(200)));  %100=1s

== matlab function SSM/StateManagement/State detection/PrechargeCheck ==
  data: uDc input; bPreChrgDone output; uDcLinkPreChrg input
function bPreChrgDone  = fcn(uDc,uDcLinkPreChrg)
%
persistent uDc_last;

if isempty(uDc_last)
    uDc_last = single(0);
end

if (uDc>uDcLinkPreChrg)&&(abs(uDc-uDc_last))<single(5) %200 to 30
    bPreChrgDone = true;
else
    bPreChrgDone = false;
end

uDc_last = uDc;

== matlab function SSM/StateManagement/State detection/FailureManage ==
  data: cntPreFailrPerm input; bRdyHiIgbtDrv input; bRdyLoIgbtDrv input; ReqPreFaiMod input; stDrvMode input; bIgbtDrvHiErr input; bIgbtDrvLoErr input; bPreFailure output; bRecovery output; bFailure output; stGateDrvFail output; bESO output; bReqFailrMod input; bReqEmgyShutOff input; flgIgrDfc input
function [bPreFailure,bRecovery,bFailure,stGateDrvFail,bESO]  =...
         fcn(cntPreFailrPerm,bRdyHiIgbtDrv,bRdyLoIgbtDrv,ReqPreFaiMod,stDrvMode,...
         bIgbtDrvHiErr,bIgbtDrvLoErr,bReqFailrMod,bReqEmgyShutOff,flgIgrDfc)
%
persistent cntFailure;
persistent cntPreFailure;
persistent stPreFailure;
persistent stGateDrvFailTmp;
persistent bESOTmp;
persistent bFailureTmp;

if isempty(cntFailure)
    cntFailure = uint8(0);
    cntPreFailure = uint8(0);
    stPreFailure = false;
    stGateDrvFailTmp = EGM.Freewheel;
    bESOTmp = false;
    bFailureTmp = false;
end

%maximum Is x 1.05
%if ((stDrvMode==ECM.Standby)||(stDrvMode==ECM.TrqCtrl)||(stDrvMode==ECM.nCtrl)||(stDrvMode==ECM.UdcCtrl)||(stDrvMode==ECM.IsCtrl))...
%    &&((Vdc>UdcMax)||(Is>IsMax)||(~bRdyHiIgbtDrv)||(~bRdyLoIgbtDrv))
if ReqPreFaiMod
    cntPreFailure = cntPreFailure + uint8(1);
    stPreFailure = true;
else
    cntPreFailure = cntPreFailure - uint8(1);
end

if (stPreFailure==true)&&(~ReqPreFaiMod)&&bRdyHiIgbtDrv&&bRdyLoIgbtDrv %maximum ASC current
    bRecovery = true;
    stPreFailure = false;
    cntFailure = cntFailure + uint8(1);
else
    bRecovery = false;
end

bPreFailure = stPreFailure;

%Failure judge
%if (cntPreFailure>uint8(5))||(cntFailure>uint8(2))...
%   ||flgFltAHiDrv||flgFltALoDrv||flgFltOC||flgFltOV||flgFltBHiDrv||flgFltBLoDrv...
%   ||flgTiOutErrAlOfsCal||(stAlOfsCal==uint8(2))||((~bVdd15Ok)&&bVdd15OkLst)
if  ((bReqFailrMod||bReqEmgyShutOff)&&flgIgrDfc)||(cntPreFailure>cntPreFailrPerm)
    bFailureTmp = true;
    
    if bReqEmgyShutOff
        bESOTmp = true;
        stGateDrvFailTmp = EGM.Shortcircuit;
    else
        if bIgbtDrvHiErr
            if bIgbtDrvLoErr
                bESOTmp = true;
                stGateDrvFailTmp = EGM.Shortcircuit;
            else
                stGateDrvFailTmp = EGM.Shortcircuit;
            end
        else
            if bIgbtDrvLoErr
                stGateDrvFailTmp = EGM.ShortcircuitTop;
            else
                stGateDrvFailTmp = EGM.Shortcircuit;
            end
        end
    end
end

if stDrvMode==ECM.Afterrun
    bESOTmp = true;
end

bFailure = bFailureTmp;  
%bFailure = false;   %used for test
stGateDrvFail = stGateDrvFailTmp;
bESO = bESOTmp;
%bESO = false; %used for test
